simulink model "RobotController3"  (R2018a)
settings: Solver=VariableStepAuto  StartTime=0.0  StopTime=500.0  RelTol=1e-3
settings Model: Creator=Carapinha  LastModifiedBy=Carapinha
settings CodeAppCC: StateflowObjectComments=on

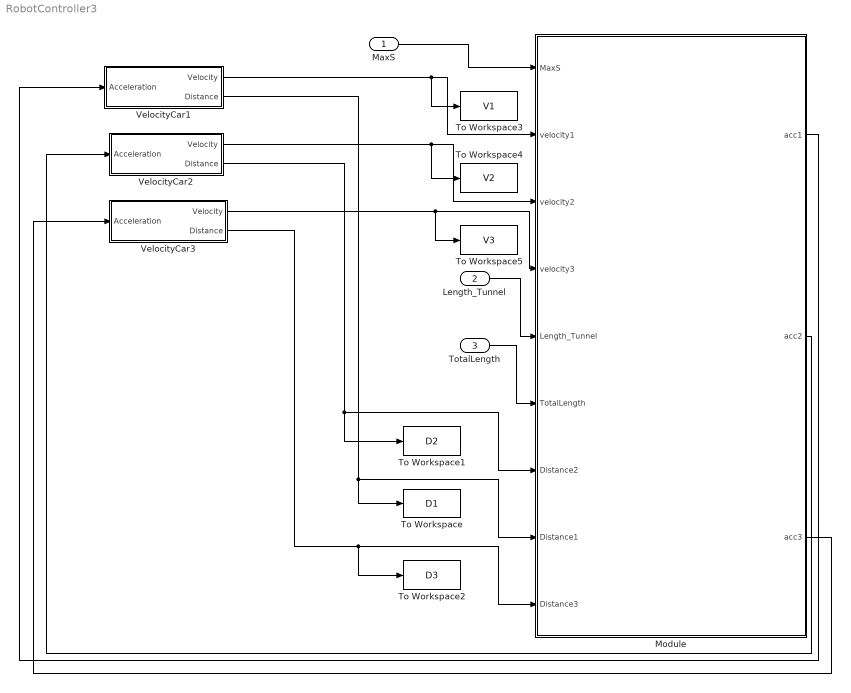
== system RobotController3 ==
  MaxS : Inport
  Length_Tunnel : Inport  Port=2
  TotalLength : Inport  Port=3
  Module : Stateflow chart  TreatAsAtomicUnit=on
  To Workspace : ToWorkspace  VariableName=D1  SaveFormat=Timeseries  SampleTime=-1
  To Workspace1 : ToWorkspace  VariableName=D2  SaveFormat=Timeseries  SampleTime=-1
  To Workspace2 : ToWorkspace  VariableName=D3  SaveFormat=Timeseries  SampleTime=-1
  To Workspace3 : ToWorkspace  VariableName=V1  SaveFormat=Timeseries  SampleTime=-1
  To Workspace4 : ToWorkspace  VariableName=V2  SaveFormat=Timeseries  SampleTime=-1
  To Workspace5 : ToWorkspace  VariableName=V3  SaveFormat=Timeseries  SampleTime=-1
  VelocityCar1 : Subsystem
  VelocityCar2 : Subsystem
  VelocityCar3 : Subsystem
  wires:
  MaxS/1 -> Module/1(MaxS)
  Module/1(acc1) -> VelocityCar1/1("Acceleration ")
  Module/2(acc2) -> VelocityCar2/1(Acceleration)
  VelocityCar1/1(Velocity) -> To Workspace3/1, Module/2(velocity1)
  VelocityCar2/1(Velocity) -> To Workspace4/1, Module/3(velocity2)
  VelocityCar3/1(Velocity) -> To Workspace5/1, Module/4(velocity3)
  Module/3(acc3) -> VelocityCar3/1(Acceleration)
  Length_Tunnel/1 -> Module/5(Length_Tunnel)
  TotalLength/1 -> Module/6(TotalLength)
  VelocityCar2/2(Distance) -> To Workspace1/1, Module/7(Distance2)
  VelocityCar1/2(Distance) -> To Workspace/1, Module/8(Distance1)
  VelocityCar3/2(Distance) -> To Workspace2/1, Module/9(Distance3)

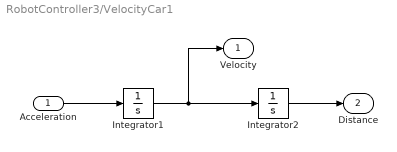
== system RobotController3/VelocityCar1 ==
  "Acceleration " : Inport
  Integrator1 : Integrator  InitialCondition=1  WrapState=on  WrappedStateUpperValue=MaxS  WrappedStateLowerValue=0
  Integrator2 : Integrator  WrapState=on  WrappedStateUpperValue=TotalLength  WrappedStateLowerValue=0
  Velocity : Outport
  Distance : Outport  Port=2
  wires:
  "Acceleration "/1 -> Integrator1/1
  Integrator1/1 -> Integrator2/1, Velocity/1
  Integrator2/1 -> Distance/1

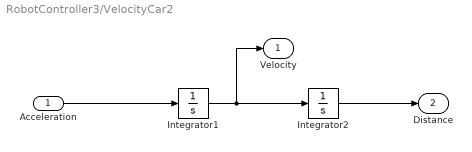
== system RobotController3/VelocityCar2 ==
  Acceleration : Inport
  Integrator1 : Integrator  InitialCondition=1  WrapState=on  WrappedStateUpperValue=MaxS  WrappedStateLowerValue=0
  Integrator2 : Integrator  WrapState=on  WrappedStateUpperValue=TotalLength  WrappedStateLowerValue=0
  Velocity : Outport
  Distance : Outport  Port=2
  wires:
  Acceleration/1 -> Integrator1/1
  Integrator1/1 -> Integrator2/1, Velocity/1
  Integrator2/1 -> Distance/1

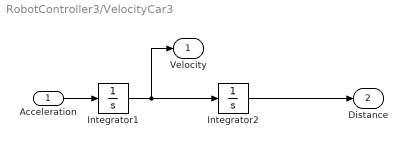
== system RobotController3/VelocityCar3 ==
  Acceleration : Inport
  Integrator1 : Integrator  InitialCondition=1  WrapState=on  WrappedStateUpperValue=MaxS  WrappedStateLowerValue=0
  Integrator2 : Integrator  WrapState=on  WrappedStateUpperValue=TotalLength  WrappedStateLowerValue=0
  Velocity : Outport
  Distance : Outport  Port=2
  wires:
  Acceleration/1 -> Integrator1/1
  Integrator1/1 -> Integrator2/1, Velocity/1
  Integrator2/1 -> Distance/1

== stateflow chart RobotController3/Module ==
  state Main
    state Robot2 [parallel]
      settings: executionOrder=3
      state move3
        entry:
        %EnterTunnel
        LeftC2 = 0;
        close2 = 0;
        Enter2 = 1;
        Stop2 = 0;
        during:
        acc2 = 0;
      state move1
        entry:
        %LeftTunnel
        LeftC2 = 1;
        close2 = 0;
        Enter2 = 0;
        Stop2 = 0;
      state move2
        entry:
        %CloseToTunnel
        LeftC2 = 0;
        close2 = 1;
        Enter2 = 0;
        Stop2 = 0;
      state Decel
        entry:
        %CriticalPoint
        LeftC2 = 0;
        close2 = 1;
        Stop2 = 0;
        Enter2 = 0;
        during:
        acc2 = -0.01;
      state Accel
        entry:
        %EnterTunnel
        LeftC2 = 0;
        close2 = 0;
        Enter2 = 1;
        Stop2 = 0;
        during:
        acc2 = 0.01;
      state Wait
        entry:
        %Stopped
        LeftC2 = 0;
        close2 = 0;
        acc2 = 0;
        Enter2 = 0;
        Stop2 = 1;
      Main.Robot2.move3 -> Main.Robot2.move1 : [Distance2 >= Length_Tunnel]
      (default) -> Main.Robot2.move1
      Main.Robot2.move1 -> Main.Robot2.move2 : [Distance2 >= 0.7*TotalLength]
      Main.Robot2.move2 -> Main.Robot2.move3 [order 1] : [Permission2 == 1]
      Main.Robot2.move2 -> Main.Robot2.Decel [order 2] : [Distance1 >= 0.9*TotalLength]
      Main.Robot2.Accel -> Main.Robot2.move3 : [velocity2 >= MaxS]
      Main.Robot2.Decel -> Main.Robot2.Accel [order 1] : [Permission2 == 1]
      Main.Robot2.Decel -> Main.Robot2.Wait [order 2] : [velocity2 <= 0]
      Main.Robot2.Wait -> Main.Robot2.Accel [order 1] : [Permission2 == 1]
      Main.Robot2.Wait -> Main.Robot2.Wait [order 2] : [Permission2 == 0]
    state Robot1 [parallel]
      settings: executionOrder=1
      state move3
        entry:
        %EnterTunnel
        LeftC = 0;
        close = 0;
        Enter = 1;
        Stop = 0;
        during:
        acc1 = 0;
      state move2
        entry:
        %CloseToTunnel
        LeftC = 0;
        close = 1;
        Enter = 0;
        Stop = 0;
      state move1
        entry:
        %LeftTunnel
        LeftC = 1;
        close = 0;
        Stop = 0;
        Enter = 0;
      state Decel
        entry:
        %CriticalPoint
        Enter = 0;
        LeftC = 0;
        close = 1;
        Stop = 0;
        during:
        acc1 = -0.01;
      state Accel
        entry:
        %EnterTunnel
        acc1 = 0.01;
        Enter = 1;
        LeftC = 0;
        close = 0;
        Stop = 0;
      state Wait
        entry:
        %Stopped
        acc1 = 0;
        Enter = 0;
        LeftC = 0;
        close = 0;
        Stop = 1;
      Main.Robot1.move3 -> Main.Robot1.move1 : [Distance1 >= Length_Tunnel]
      (default) -> Main.Robot1.move1
      Main.Robot1.move1 -> Main.Robot1.move2 : [Distance1 >= 0.7*TotalLength]
      Main.Robot1.move2 -> Main.Robot1.move3 [order 1] : [Permission1 == 1]
      Main.Robot1.move2 -> Main.Robot1.Decel [order 2] : [Distance1 >= 0.9*TotalLength]
      Main.Robot1.Accel -> Main.Robot1.move3 : [velocity1 >= MaxS]
      Main.Robot1.Decel -> Main.Robot1.Accel [order 1] : [Permission1 == 1]
      Main.Robot1.Decel -> Main.Robot1.Wait [order 2] : [velocity1 <= 0]
      Main.Robot1.Wait -> Main.Robot1.Accel [order 1] : [Permission1 == 1]
      Main.Robot1.Wait -> Main.Robot1.Wait [order 2] : [Permission1 == 0]
    state Robot3 [parallel]
      settings: executionOrder=4
      state move3
        entry:
        %EnterTunnel
        LeftC3 = 0;
        close3 = 0;
        Enter3 = 1;
        Stop3 = 0;
        during:
        acc3 = 0;
      state move1
        entry:
        %LeftTunnel
        LeftC3 = 1;
        close3 = 0;
        Enter3 = 0;
        Stop3 = 0;
      state move2
        entry:
        %CloseToTunnel
        LeftC3 = 0;
        close3 = 1;
        Enter3 = 0;
        Stop3 = 0;
      state Decel
        entry:
        %CriticalPoint
        LeftC3 = 0;
        close3 = 1;
        Enter3 = 0;
        Stop3 = 0;
        during:
        acc3 = -0.01;
      state Accel
        entry:
        %EnterTunnel
        LeftC3 = 0;
        close3 = 0;
        Enter3 = 1;
        Stop3 = 0;
        during:
        acc3 = 0.01;
      state Wait
        entry:
        %Stopped
        LeftC3 = 0;
        close3 = 0;
        Enter3 = 0;
        Stop3 = 1;
        acc3 = 0;
      Main.Robot3.move3 -> Main.Robot3.move1 : [Distance3 >= Length_Tunnel]
      (default) -> Main.Robot3.move1
      Main.Robot3.move1 -> Main.Robot3.move2 : [Distance3 >= 0.7*TotalLength]
      Main.Robot3.move2 -> Main.Robot3.move3 [order 1] : [Permission3 == 1]
      Main.Robot3.move2 -> Main.Robot3.Decel [order 2] : [Distance3 >= 0.9*TotalLength]
      Main.Robot3.Accel -> Main.Robot3.move3 : [velocity3 >= MaxS]
      Main.Robot3.Decel -> Main.Robot3.Accel [order 1] : [Permission3 == 1]
      Main.Robot3.Decel -> Main.Robot3.Wait [order 2] : [velocity3 <= 0]
      Main.Robot3.Wait -> Main.Robot3.Accel [order 1] : [Permission3 == 1]
      Main.Robot3.Wait -> Main.Robot3.Wait [order 2] : [Permission3 == 0]
    state Controller [parallel]
      settings: executionOrder=2
      state FirstCar
        entry:
        Permission1 = 1;
        Permission2 = 0;
        Permission3 = 0;
      state ThirdCar2
      state SecCar
        entry:
        Permission1 = 0;
        Permission2 = 1;
        Permission3 = 0;
      state SecCar1
      state RobotState
      state ThirdCar1
      state ThirdCar
        entry:
        Permission1 = 0;
        Permission2 = 0;
        Permission3 = 1;
      FirstCar -> RobotState : [LeftC == 1]
      ThirdCar2 -> FirstCar : [Enter2 == 0  && Enter3 == 0]
      RobotState -> ThirdCar2 [order 2] : [close == 1 || Enter == 1]
      (default) -> RobotState
      RobotState -> SecCar1 [order 3] : [close2 == 1 || Enter2 == 1]
      SecCar1 -> SecCar : [Enter == 0 && Enter3 == 0]
      SecCar -> RobotState : [LeftC2 == 1]
      RobotState -> ThirdCar1 [order 1] : [close3 == 1 || Enter3 == 1]
      ThirdCar -> RobotState : [LeftC3 == 1]
      ThirdCar1 -> ThirdCar : [Enter == 0 && Enter2 == 0]
  (default) -> Main
  data: MaxS input; Permission1 local =0; Permission2 local =0; Decel local; Accel local; acc1 output; acc2 output; velocity1 input; velocity2 input; velocity3 input; acc3 output; close3 local; Enter3 local; LeftC3 local; Stop3 local; Permission3 local =0; Length_Tunnel input; TotalLength input; LeftC local; close local; cp local; LeftC2 local; cp2 local; Enter local; Stop local; close2 local; Stop2 local; Enter2 local; cp3 local; Distance2 input; Distance1 input; Distance3 input
